simulink model "ALFlight3"  (R2019a)
settings: Solver=VariableStepAuto  StartTime=0.0  StopTime=100  RelTol=1e-3
InitFcn:
  | Ts=.05
  | load('goodMPC.mat')
  | %load('fault2mpc.mat')
  | global counts
  | counts=0
  | 
  | An=[-0.0220400000000000,0.00142200000000000,0,-32.1700000000000,0,0,0,0,0,0;-0.0575900000000000,-0.394300000000000,871,0,0,0,0,0,0,0;-9.50000000000000e-05,-0.00179300000000000,-0.546800000000000,0,0,0,0,0,0,0;0,0,1,0,0,0,0,0,0,0;0,0,0,0,-0.0639900000000000,0,-1,0.0369100000000000,0,0;0,0,0,0,-2.11100000000000,-0.504800000000000,0.193000000000000,0,0,0;0,0,0,0,0.773200000000000,0.0108700000000000,-0.179400000000000,0,0,0;0,0,0,0,0,1,0,0,0,0;0,0,0,0,0,0,1,0,0,0;0,1,0,0,0,0,0,0,0,0]
  | Bn=[0,1.91000000000000e-05,0,0;-18.5800000000000,0,0,0;-1.20000000000000,0,0,0;0,0,0,0;0,0,0,0.00839000000000000;0,0,0.184800000000000,0.105600000000000;0,0,-0.00869900000000000,-0.459100000000000;0,0,0,0;0,0,0,0;0,0,0,0]
  | 
  | load('finalWorkspace.mat')
  |  set_param('ALFlight3/ConstantA','Value','An')
  |  set_param('ALFlight3/ConstantB','Value','Bn')
model workspace (MAT data in the model file):
  MCOS : class17 (value not decoded)
values from neighbouring files (symbols this model uses):
  AfU = [-0.0194355650403 0 0.00129160400584 0 0 0 0 0 0 0 0.0910789295705 -0.529233298764 ... (100 elements, 10x10)]    [finalWorkspace.mat]
  BfU = [0 -0.0292332987635 -0.465820206007 0 0 0 0 0 0 0 4.775e-06 0 ... (40 elements, 10x4)]    [finalWorkspace.mat]
  Cn = [1 0 0 0 0 0 0 0 0 0 0 0 ... (40 elements, 4x10)]    [UpdatedWorkspace.mat]    (also in current2.mat; finalWorkspace.mat)
  Dn = [0 0 0 0 0 0 0 0 0 0 0 0 ... (16 elements, 4x4)]    [UpdatedWorkspace.mat]    (also in current2.mat; finalWorkspace.mat)
  p = 15    [calcVar.m]    (also in chanceConstraintProgramming4.m = [norminv(.505),norminv(.6),norminv(.7),norminv(.8),norminv(.; dynamicsEst.m)
undefined symbols (not defined in the file or in its folder): Earth, iA, lastPcov, lastu, lastx, MDscale, MVscale, nCC, nu, nud, nv, ny, nym, RMVscale, RYscale, ts, uoff, WGS84, xoff, Yscale
libraries: mpcsigdimcheck_private x26, simulink_extras x3, aerolibtransform2 x1, aerolibfltsims x1, commchan3 x1, aerolibanimutils x1
(part 2 of 2)

== matlab function ALFlight3/Plant/MATLAB Function ==
  data: nextState output; state input; y output; action input; Ts input; time input; currentState data_store_memory; counts data_store_memory; Damage data_store_memory
function [nextState,y] = fcn2(state, action,Ts,time)
global currentState
global Damage
coder.extrinsic('evalin')
coder.extrinsic('assignin')
Anominal=[-0.0220400000000000,0.00142200000000000,0,-32.1700000000000,0,0,0,0,0,0,0;
    -0.0575900000000000,-0.394300000000000,871,0,0,0,0,0,0,0,0;
    -9.50000000000000e-05,-0.00179300000000000,-0.546800000000000,0,0,0,0,0,0,0,0;
    0,0,1,0,0,0,0,0,0,0,0;
    0,0,0,0,-0.0639900000000000,0,-1,0.0369100000000000,0,0,0;
    0,0,0,0,-2.11100000000000,-0.504800000000000,0.193000000000000,0,0,0,0;
    0,0,0,0,0.773200000000000,0.0108700000000000,-0.179400000000000,0,0,0,0;
    0,0,0,0,0,1,0,0,0,0,0;
    0,0,0,0,0,0,1,0,0,0,0;
    1,0,0,0,0,0,0,0,0,0,0;
    0,1,0,0,0,0,0,0,0,0,0];
Bnominal=[0,1.91000000000000e-05,0,0;
    -18.5800000000000,0,0,0;
    -1.20000000000000,0,0,0;
    0,0,0,0;
    0,0,0,0.00839000000000000;
    0,0,0.184800000000000,0.105600000000000;
    0,0,-0.00869900000000000,-0.459100000000000;
    0,0,0,0;
    0,0,0,0;
    0,0,0,0;
    0,0,0,0];

Afault2=[-0.0220400000000000,0.00142200000000000,0,-32.1700000000000,0,0,0,0,0,0,0;
    -0.0575900000000000,-0.394300000000000,871,0,0,0,0,0,0,0,0;
    -9.50000000000000e-05,-0.00179300000000000,-0.546800000000000,0,0,0,0,0,0,0,0;
    0,0,1,0,0,0,0,0,0,0,0;
    0,0,0,0,0,-0.00110800000000000,-1,0.0369100000000000,0,0,0;
    0,0,0,0,-1.23500000000000,-0.481800000000000,0.0891100000000000,0,0,0,0;
    0,0,0,0,0,-0.0519300000000000,0,0,0,0,0;
    0,0,0,0,0,1,0,0,0,0,0;
    0,0,0,0,0,0,1,0,0,0,0;
    1,0,0,0,0,0,0,0,0,0,0;
    0,1,0,0,0,0,0,0,0,0,0];
Bfault2=[0,1.91000000000000e-05,0,0;
    -18.5800000000000,0,0,0;
    -1.20000000000000,0,0,0;
    0,0,0,0;
    0,0,0,0;
    0,0,0.187900000000000,0;
    0,0,0,0;
    0,0,0,0;
    0,0,0,0;
    0,0,0,0;
    0,0,0,0];

Afault1_2=[-0.0777422601610909,0.364315718281914,0,-49.5311012194985,0,0,0,0,0,0,0;
    0,-2.11693319505418,-8.082029025490,0,0,0,0,0,0,0,0;
    0.00516641602336364,-3.5543885272319,-2.926680000000,-2.37481704217243,0,0,0,0,0,0,0;
    0,0,1,0,0,0,0,0,0,0,0;
    0,0,0,0,-1.73568157299046,-0.00695689900121296,-246.715568807515,49.5311012194985,0,0,0;
    0,0,32.90144280000,31.3713331270978,-0.0210854784922154,-0.00633571574984461,0.00174212652554297,0,0,0,0;
    0,0,0,13.2100000000000,0.0233794202315124,-4.26083552968259e-05,-0.00576851579403181,0,0,0,0;
    0,0,0,0,0,1,0.0479459770467924,0,0,0,0;
    0,0,0,0,0,0,1,0,0,0,0;
    1,0,0,0,0,0,0,0,0,0,0;
    0,1,0,0,0,0,0,0,0,0,0]*.25
Bfault1_2=[0,0,0,0;
    -.11693319505418,0,0,0;
    -1.863280824027,0,0,0;
    0,0,0,0;
    0,0,0,-0.00412083182815909;
    0,0,0.00602442242634726,0.00602442242634726;
    0,0,0,-0.0221156677865658;
    0,0,0,0;0,0,0,0;0,0,0,0;0,0,0,0]*.25
 
Afault1=[-0.00470000000000000,-0.0107700000000000,0,-623300,0,0,0,0,0,0,0;
     -0.310000000000000,-0.253000000000000,16780000,-28300,0,0,0,0,0,0,0;
     0,0,-157900,264.600000000000,0,0,0,0,0,0,0;
     0,0,1,0,0,0,0,0,0,0,0;
     0,0,0,0,-0.0470000000000000,0,-16890000,620000,0,0,0;
     0,0,463000,-7797,-0.00160000000000000,-0.201300000000000,0.105500000000000,0,0,0,0;
     0,0,0,171900,0.000570000000000000,-0.00650000000000000,-157900,5833,0,0,0;
     0,0,0,0,0,1,0.0454100000000000,0,0,0,0;
     0,0,0,0,0,0,1,0,0,0,0;
     1,0,0,0,0,0,0,0,0,0,0;
     0,871,0,0,0,0,0,0,0,0,0];
 Bfault1=[0,0,0,0;
     13.3300000000000,0,0,0;
     -0.914700000000000,0,0,0;
     0,0,0,0;
     0,0,0,5.37700000000000;
     0,0,0.0670800000000000,0.0762900000000000;
     0,0,13.3200000000000,-0.289500000000000;
     0,0,0,0;
     0,0,0,0;
     0,0,0,0;
     0,0,0,0];
 
 
 Afault3=[-0.0220400000000000,0.00142200000000000,0,-32.1700000000000,0,0,0,0,0,0,0;-0.0575900000000000,-0.394300000000000,871,0,0,0,0,0,0,0,0;-9.50000000000000e-05,-0.00179300000000000,-0.546800000000000,0,0,0,0,0,0,0,0;0,0,1,0,0,0,0,0,0,0,0;0,0,0,0,-0.0639900000000000,0,-1,0.0369100000000000,0,0,0;0,0,0,0,-2.11100000000000,-0.504800000000000,0.193000000000000,0,0,0,0;0,0,0,0,0.773200000000000,0.0108700000000000,-0.179400000000000,0,0,0,0;0,0,0,0,0,1,0,0,0,0,0;0,0,0,0,0,0,1,0,0,0,0;1,0,0,0,0,0,0,0,0,0,0;0,1,0,0,0,0,0,0,0,0,0]
Bfault3=[0,1.91000000000000e-05,0,0;
    -18.5800000000000,0,0,0;
    -1.20000000000000,0,0,0;
    0,0,0,0;
    0,0,0,0.00839000000000000;
    0,0,0,0.105600000000000;
    0,0,0,-0.459100000000000;
    0,0,0,0;
    0,0,0,0;
    0,0,0,0;
    0,0,0,0]
 
 % C=[1,0,0,0,0,0,0,0,0,0,0;
%     0,0,0,1,0,0,0,0,0,0,0;
%     0,0,0,0,0,0,0,1,0,0,0;
%     0,0,0,0,0,0,0,0,1,0,0;
%     0,0,0,0,0,0,0,0,0,1,0;
%     0,0,0,0,0,0,0,0,0,0,1]
 %y=zeros(6,1);
deltaS=zeros(11,1)
if Damage==1
    ADamage=Afault1_2
    BDamage=Bfault1_2
    A=evalin('base','Af1')
    assignin('base','AfU',A)
    B=evalin('base','Bf1')
    assignin('base','BfU',B)
elseif Damage==2
    ADamage=Afault2
    BDamage=Bfault2 
    A=evalin('base','Af2')
    assignin('base','AfU',A)
    B=evalin('base','Bf2')
    assignin('base','BfU',B)
elseif Damage==3
    ADamage=Afault3
    BDamage=Bfault3
    A=evalin('base','Af3')
    assignin('base','AfU',A)
    B=evalin('base','Bf3')
    assignin('base','BfU',B)
else
    ADamage=Afault2
    BDamage=Bfault2
    A=evalin('base','Af2')
    assignin('base','AfU',A)
    B=evalin('base','Bf2')
    assignin('base','BfU',B)
end
    
 if time<10
     deltaS=Anominal*state*Ts+Bnominal*action*Ts;
     nextState=deltaS+state
    y=nextState
 else
     deltaS=ADamage*state*Ts+BDamage*action*Ts
     nextState=deltaS+state
     y=nextState
 end
 currentState=y
end

== matlab function ALFlight3/Error/MATLAB Function2 ==
  data: error input; counts data_store_memory
function fcn(error)
global counts
if error>.1
counts=counts+1
end

== matlab function ALFlight3/MATLAB Function3 ==
  data: outputs input; counts data_store_memory; savedOutputs data_store_memory
function saveDataOutputs(outputs)
global savedOutputs
global counts
if counts>0
savedOutputs(:,counts)=outputs
end
x=savedOutputs

== matlab function ALFlight3/State space model ==
  data: state input; nextState output; action input; Ts input; time input; action output; y output
function [nextState,action,y] = fcn(state, action, Ts,time)
Anominal=[-0.0220400000000000,0.00142200000000000,0,-32.1700000000000,0,0,0,0,0,0,0,0;-0.0575900000000000,-0.394300000000000,871,0,0,0,0,0,0,0,0,0;-9.50000000000000e-05,-0.00179300000000000,-0.546800000000000,0,0,0,0,0,0,0,0,0;0,0,1,0,0,0,0,0,0,0,0,0;0,0,0,0,-0.0639900000000000,0,-1,0.0369100000000000,0,0,0,0;0,0,0,0,-2.11100000000000,-0.504800000000000,0.193000000000000,0,0,0,0,0;0,0,0,0,0.773200000000000,0.0108700000000000,-0.179400000000000,0,0,0,0,0;0,0,0,0,0,1,0,0,0,0,0,0;0,0,0,0,0,0,1,0,0,0,0,0;1,0,0,0,0,0,0,0,0,0,0,0;0,1,0,0,0,0,0,0,0,0,0,0;0,0,0,0,0,0,0,0,0,0,0,0]
Bnominal=[0,1.91000000000000e-05,0,0;-18.5800000000000,0,0,0;-1.20000000000000,0,0,0;0,0,0,0;0,0,0,0.00839000000000000;0,0,0.184800000000000,0.105600000000000;0,0,-0.00869900000000000,-0.459100000000000;0,0,0,0;0,0,0,0;0,0,0,0;0,0,0,0;0,0,0,0]

Afault2=[-0.0220400000000000,0.00142200000000000,0,-32.1700000000000,0,0,0,0,0,0,0;
    -0.0575900000000000,-0.394300000000000,871,0,0,0,0,0,0,0,0;
    -9.50000000000000e-05,-0.00179300000000000,-0.546800000000000,0,0,0,0,0,0,0,0;
    0,0,1,0,0,0,0,0,0,0,0;
    0,0,0,0,0,-0.00110800000000000,-1,0.0369100000000000,0,0,0;
    0,0,0,0,-1.23500000000000,-0.481800000000000,0.0891100000000000,0,0,0,0;
    0,0,0,0,0,-0.0519300000000000,0,0,0,0,0;
    0,0,0,0,0,1,0,0,0,0,0;
    0,0,0,0,0,0,1,0,0,0,0;
    1,0,0,0,0,0,0,0,0,0,0;
    0,1,0,0,0,0,0,0,0,0,0];
Bfault2=[0,1.91000000000000e-05,0,0;
    -18.5800000000000,0,0,0;
    -1.20000000000000,0,0,0;
    0,0,0,0;
    0,0,0,0;
    0,0,0.187900000000000,0;
    0,0,0,0;
    0,0,0,0;
    0,0,0,0;
    0,0,0,0;
    0,0,0,0];
     
 Afault1=[-0.00470000000000000,-0.0107700000000000,0,-623300,0,0,0,0,0,0,0;
     -0.310000000000000,-0.253000000000000,16780000,-28300,0,0,0,0,0,0,0;
     0,0,-157900,264.600000000000,0,0,0,0,0,0,0;
     0,0,1,0,0,0,0,0,0,0,0;
     0,0,0,0,-0.0470000000000000,0,-16890000,620000,0,0,0;
     0,0,463000,-7797,-0.00160000000000000,-0.201300000000000,0.105500000000000,0,0,0,0;
     0,0,0,171900,0.000570000000000000,-0.00650000000000000,-157900,5833,0,0,0;
     0,0,0,0,0,1,0.0454100000000000,0,0,0,0;
     0,0,0,0,0,0,1,0,0,0,0;
     1,0,0,0,0,0,0,0,0,0,0;
     0,1,0,0,0,0,0,0,0,0,0];
 Bfault1=[0,0,0,0;
     13.3300000000000,0,0,0;
     -0.914700000000000,0,0,0;
     0,0,0,0;
     0,0,0,5.37700000000000;
     0,0,0.0670800000000000,0.0762900000000000;
     0,0,13.3200000000000,-0.289500000000000;
     0,0,0,0;
     0,0,0,0;
     0,0,0,0;
     0,0,0,0];
C=[1,0,0,0,0,0,0,0,0,0,0,0;0,0,0,1,0,0,0,0,0,0,0,0;0,0,0,0,0,0,0,1,0,0,0,0;0,0,0,0,0,0,0,0,1,0,0,0;0,0,0,0,0,0,0,0,0,1,0,0;0,0,0,0,0,0,0,0,0,0,1,0]
y=zeros(6,1);
deltaS=zeros(12,1)
 if time<20
     deltaS=Anominal*state*.05+Bnominal*action*.05;
    nextState=(deltaS+state);
    y=C*nextState;
 else
     nextState=zeros(12,1)
%     deltaS=Afault2*state*Ts+Bfault2*action*Ts;
%     nextState=(deltaS+state);
%     y=C*nextState;
end
end

== matlab function ALFlight3/Switch /MATLAB Function4 ==
  data: a output; actionMPC input; actionAL input; counts data_store_memory; uncertainty data_store_memory; useMPC data_store_memory; ABestGuess data_store_memory
function a = switching(actionMPC,actionAL)
coder.extrinsic('evalin')
coder.extrinsic('assignin')
coder.extrinsic('set_param')
global counts
global uncertainty
global useMPC
global ABestGuess

Anominal=[-0.0220400000000000,0.00142200000000000,0,-32.1700000000000,0,0,0,0,0,0,0;
    -0.0575900000000000,-0.394300000000000,871,0,0,0,0,0,0,0,0;
    -9.50000000000000e-05,-0.00179300000000000,-0.546800000000000,0,0,0,0,0,0,0,0;
    0,0,1,0,0,0,0,0,0,0,0;
    0,0,0,0,-0.0639900000000000,0,-1,0.0369100000000000,0,0,0;
    0,0,0,0,-2.11100000000000,-0.504800000000000,0.193000000000000,0,0,0,0;
    0,0,0,0,0.773200000000000,0.0108700000000000,-0.179400000000000,0,0,0,0;
    0,0,0,0,0,1,0,0,0,0,0;
    0,0,0,0,0,0,1,0,0,0,0;
    1,0,0,0,0,0,0,0,0,0,0;
    0,1,0,0,0,0,0,0,0,0,0];
Bnominal=[0,1.91000000000000e-05,0,0;
    -18.5800000000000,0,0,0;
    -1.20000000000000,0,0,0;
    0,0,0,0;
    0,0,0,0.00839000000000000;
    0,0,0.184800000000000,0.105600000000000;
    0,0,-0.00869900000000000,-0.459100000000000;
    0,0,0,0;
    0,0,0,0;
    0,0,0,0;
    0,0,0,0];



a=actionMPC;
if counts>3 && ~useMPC
    a=actionAL;
end
if uncertainty<.1
    useMPC=true
    
    
    Af=ABestGuess(5:15,:)*Anominal
    Af(abs(Af)<8e-5)=0
    AfU=Af([1 2 3 4 5 6 7 8 9 11],[1 2 3 4 5 6 7 8 9 11])
    Bf= ABestGuess(1:4,:)'+ABestGuess(5:15,:)'*Bnominal
    Bf(abs(Bf)<1e-5)=0
    BfU=Bf([1 2 3 4 5 6 7 8 9 11],:)

    Af2=evalin('base','Af2')
    Bf2=evalin('base','Bf2')
    
    
    set_param('ALFlight3/ConstantA','Value','AfU')
    set_param('ALFlight3/ConstantB','Value','BfU')

end
%     fault1MPC.Model.Plant.A=A
%     fault1MPC.Model.Plant.B=B
%     
%     fault2MPC.Model.Plant.A=A
%     fault2MPC.Model.Plant.B=B
%     
%     fault3MPC.Model.Plant.A=A
%     fault3MPC.Model.Plant.B=B
% set_param('testMPC/MPCController1','mpcobj','fault2MPC')

% a=actionMPC;
% if time>1000
%     a=actionAL;
% end

== matlab function ALFlight3/MATLAB Function5 ==
  data: inputs input; savedInputs data_store_memory; counts data_store_memory
function saveDataInputs(inputs)
global savedInputs
global counts
if counts>0
savedInputs(:,counts)=inputs
end
x=savedInputs

== matlab function ALFlight3/Update Plant Model ==
  data: Ac input; Bc input; Cc input; Dc input; u input; A output size=[10,10]; x input size=[11,1]; B output size=[10,4]; C output size=[4,10]; D output size=[4,4]; u output; Y output size=[4,1]; X output size=[10,1]; DX output size=[10,1]
function [A,B,C,D,u,Y,X,DX] = fcn(Ac,Bc,Cc,Dc,u,x)
% Sample time
Ts = 0.05;
x=[x(1:9);x(11)]
% Model parameters


% Continuous-time model
Ac = Ac
Bc =  Bc  
Cc = Cc
Dc = Dc

% Generate discrete-time model
nx = size(Ac,1);
nu = size(Bc,2);
M = expm([[Ac Bc]*Ts; zeros(nu,nx+nu)]);
A = M(1:nx,1:nx);
B = M(1:nx,nx+1:nx+nu);
C = Cc;
D = Dc;

% Nominal conditions for discrete-time plant
X = x;
U = u;
Y = C*x + D*u;
DX = A*x+B*u-x;

== matlab function ALFlight3/Adaptive MPC Controller/MPC/optimizer/FixedHorizonOptimizer ==
  settings: updateMethod=DISCRETE  sampleTime=ts
  data: xk1 output BlockDataType; xk input BlockDataType; old_u input BlockDataType; ym input BlockDataType; ref input BlockDataType; md input BlockDataType; umin input BlockDataType; umax input BlockDataType; ymin input BlockDataType; ymax input BlockDataType; E input BlockDataType; F input BlockDataType; G input BlockDataType; S input BlockDataType; switch_in input BlockDataType; ext_mv input BlockDataType; MVtarget input BlockDataType; isQP parameter boolean; nx parameter BlockDataType; nxp parameter BlockDataType; nup parameter BlockDataType; nu parameter BlockDataType; ny parameter BlockDataType; degrees parameter BlockDataType; Hinv parameter BlockDataType; Kx parameter BlockDataType; Ku1 parameter BlockDataType; Kut parameter BlockDataType; Kr parameter BlockDataType; Kv parameter BlockDataType; Mlim parameter BlockDataType; Mx parameter BlockDataType; Mu1 parameter BlockDataType; Mv parameter BlockDataType; z_degrees parameter BlockDataType; utarget parameter BlockDataType; p parameter BlockDataType; maxiter parameter BlockDataType; CustomSolver parameter boolean; CustomSolverCodeGen parameter boolean; UseWarmStart parameter boolean; UseSuboptimalSolution parameter boolean; nxQP parameter BlockDataType; openloopflag parameter boolean; no_umin parameter BlockDataType; no_umax parameter BlockDataType; no_ymin parameter BlockDataType; no_ymax parameter BlockDataType; switch_inport parameter BlockDataType; no_switch parameter BlockDataType; enable_value parameter BlockDataType; return_cost parameter BlockDataType; H parameter BlockDataType; return_mvseq parameter BlockDataType; return_xseq parameter BlockDataType; return_ovseq parameter BlockDataType; Linv parameter BlockDataType; Ac parameter BlockDataType; ywt input BlockDataType; uwt input BlockDataType; duwt input BlockDataType; rhoeps input BlockDataType; isLTV parameter boolean; a input BlockDataType; b input BlockDataType; c input BlockDataType; d input BlockDataType; U input BlockDataType; Y input BlockDataType; X input BlockDataType; DX input BlockDataType; Pk input BlockDataType; iA input boolean; u output BlockDataType; cost output BlockDataType; useq output BlockDataType; xseq output BlockDataType; yseq output BlockDataType; status output BlockDataType; xest output BlockDataType; Pk1 output BlockDataType; no_ywt parameter BlockDataType; no_uwt parameter BlockDataType; no_duwt parameter BlockDataType; no_rhoeps parameter BlockDataType; Wy parameter BlockDataType; Wdu parameter BlockDataType; Jm parameter BlockDataType; SuJm parameter BlockDataType; Su1 parameter BlockDataType; Sx parameter BlockDataType; Hv parameter BlockDataType; Wu parameter BlockDataType; I1 parameter BlockDataType; iAout output boolean; A parameter BlockDataType; C parameter BlockDataType; B parameter BlockDataType; D parameter BlockDataType; Cid parameter BlockDataType; Did parameter BlockDataType; Mrows parameter BlockDataType; nCC parameter BlockDataType; Ecc parameter BlockDataType; Fcc parameter BlockDataType; Scc parameter BlockDataType; Gcc parameter BlockDataType; nv parameter BlockDataType; no_md parameter BlockDataType; no_ref parameter BlockDataType; no_uref parameter BlockDataType; no_mv parameter BlockDataType; RYscale parameter BlockDataType; RMDscale parameter BlockDataType; myindex parameter BlockDataType; xoff parameter BlockDataType; CustomEstimation parameter boolean; mvindex parameter BlockDataType; mdindex parameter BlockDataType; unindex parameter BlockDataType; nxid parameter BlockDataType; Uscale parameter BlockDataType; Yscale parameter BlockDataType; uoff parameter BlockDataType; voff parameter BlockDataType; yoff parameter BlockDataType; myoff parameter BlockDataType; no_cc parameter BlockDataType
function [xk1, u, cost, useq, xseq, yseq, status, xest, Pk1, iAout] = fcn(...
            xk, old_u, ym, ref, md, umin, umax, ymin, ymax, E, F, G, S,...
            switch_in, ext_mv, MVtarget, isQP, nx, nxp, nup, ...
            nu, ny, degrees, Hinv, Kx, Ku1, Kut, Kr, Kv, Mlim, ...
            Mx, Mu1, Mv, z_degrees, utarget, p, maxiter, ...
            CustomSolver, CustomSolverCodeGen, UseWarmStart, UseSuboptimalSolution, nxQP, openloopflag, ...
            no_umin, no_umax, no_ymin, no_ymax, switch_inport, no_switch, enable_value, ...
            return_cost, H, return_mvseq, return_xseq, return_ovseq, Linv, Ac, ...
            ywt, uwt, duwt, rhoeps, isLTV, a, b, c, d, U, Y, X, DX, Pk, iA, ...
            no_ywt, no_uwt, no_duwt, no_rhoeps,...
            Wy, Wdu, Jm, SuJm, Su1, Sx, Hv, Wu, I1, ...
            A, C, B, D, Cid, Did, Mrows, nCC, Ecc, Fcc, Scc, Gcc, ...
            nv, no_md, no_ref, no_uref, no_mv, RYscale, RMDscale, myindex, ...
            xoff, CustomEstimation, mvindex, mdindex, unindex, nxid, Uscale, Yscale, uoff, voff, yoff, myoff, no_cc)
%#codegen
coder.extrinsic('mpcblock_optimizer_double_mex');
coder.extrinsic('mpcblock_optimizer_single_mex');
coder.extrinsic('mpcblock_refmd_double_mex');
coder.extrinsic('mpcblock_refmd_single_mex');

% Constants
isSimulation = coder.target('Sfun') && ~coder.target('RtwForRapid') && ~coder.target('RtwForSim');
isAdaptive = ~isLTV; % isLTV=true forces isAdaptive=false
isDouble = isa(ref,'double');
if isDouble
    DataType = 'double';
else
    DataType = 'single';
end
ZERO = zeros('like',ref);
ONE = ones('like',ref);
hasMD = nv>1;

% Pre-allocate all the MEX block outputs for the simulation mode
%#ok<*NASGU>
if isSimulation
    rseq = zeros(p*ny,1,'like',ref); %#ok<*NASGU>
    vseq = zeros((p+1)*nv,1,'like',ref);
    v = zeros(nv,1,'like',ref);
    xk1 = zeros(nx,1,'like',ref);
    u = zeros(nu,1,'like',ref);
    cost = ZERO;
    useq = zeros(p+1,nu,'like',ref); %#ok<*PREALL>
    status = ONE;
    xest = zeros(nx,1,'like',ref);
    iAout = iA;
end

% Model update
nym = length(myindex);
ai=zeros(nxp,nxp,'like',ref);
bi=zeros(nxp,nup,'like',ref);
ci=zeros(ny,nxp,'like',ref);
di=zeros(ny,nup,'like',ref);

ai(:,:)=a(:,:,1);
bi(:,:)=b(:,:,1);
ci(:,:)=c(:,:,1);
di(:,:)=d(:,:,1);

% Allocate matrices. Must allocate 3D matrix also in Adaptive case,
% otherwise EML code does not compile.
Bu=zeros(nx,nu,p+1,'like',ref);
Bv=zeros(nx,nv,p+1,'like',ref);
Dv=zeros(ny,nv,p+1,'like',ref);
Dvm=zeros(nym,nv,p+1,'like',ref);
Cm=zeros(nym,nx,p+1,'like',ref);
if ~isLTV
    % Adaptive
    [A(:,:,1),C(:,:,1),Bu(:,:,1),Bv(:,:,1),Cm(:,:,1),Dv(:,:,1),Dvm(:,:,1),Qk,Rk,Nk] = mpc_plantupdate(...
        ai,bi,ci,di,A(:,:,1),B(:,:,1),C(:,:,1),D(:,:,1),mvindex,mdindex,unindex,nxp,nup,ny,nv,nxid, ...
        myindex,Uscale,Yscale,Cid,Did);
else
    % Retrieve LTV model
    for i=1:p+1
        ai(1:nxp,1:nxp)=a(:,:,i);
        bi(1:nxp,1:nup)=b(:,:,i);
        ci(1:ny,1:nxp)=c(:,:,i);
        di(1:ny,1:nup)=d(:,:,i);
        [A(:,:,i),C(:,:,i),Bu(:,:,i),Bv(:,:,i),Cm(:,:,i),Dv(:,:,i),Dvm(:,:,i),Qk,Rk,Nk] =...
            mpc_plantupdate(ai,bi,ci,di,A(:,:,i),B(:,:,i),C(:,:,i),D(:,:,i),mvindex,mdindex,unindex,nxp,nup,ny,nv,nxid, ...
            myindex,Uscale,Yscale,Cid,Did);
    end
end

% Offset update together with Mlim, utarget, Bv and Dv values
[Mlim, utarget, uoff, voff, yoff, myoff, xoff, Bv, Dv] = ...
    mpc_updateFromNominal(isAdaptive,isQP,p,Mlim,Mrows,...
       U,Uscale,uoff,mvindex,voff,mdindex,utarget,nu,nv-1,...
       Y,Yscale,yoff,myoff,myindex,ny,...
       X,xoff,nxp,DX,A,Bu,Bv,C,Dv,nCC);

% Remove last u offset
old_u = old_u - uoff;       

% Get reference and MD signals -- accounting for previewing
if isSimulation
    if isDouble
        [rseq, vseq, v] = mpcblock_refmd_double_mex(ref,md,nv,ny,p,yoff,voff,no_md,no_ref,openloopflag, RYscale, RMDscale);
    else
        [rseq, vseq, v] = mpcblock_refmd_single_mex(ref,md,nv,ny,p,yoff,voff,no_md,no_ref,openloopflag, RYscale, RMDscale);        
    end
else
    % When doing code generation, use M code directly
    [rseq, vseq, v] = mpcblock_refmd(ref,md,nv,ny,p,yoff,voff,no_md,no_ref,openloopflag, RYscale, RMDscale);
end

% External MV override.  
% NOTE: old_u and ext_mv input signals are dimensionless and offset-free.
if no_mv==ONE
    % no external mv: old_u is the optimal u[k-1] from last_mv
    delmv = zeros(nu,1,'like',ref);
else
    % has external mv: old_u is the external u[k-1]
    ext_mv = ext_mv - uoff;     % bias correction
    delmv = ext_mv - old_u;
    old_u = ext_mv;
end

% Obtain x[k|k]
xk = xk - xoff;     % Remove offset
if CustomEstimation==ONE
    % Input is x(k|k)
    xest = xk;
else
    % Calculate gain matrices, and perform measurement update.
    Kinv = eye(nym,'like',ref)/(Cm(:,:,1)*Pk*Cm(:,:,1)' + Rk);
    L = (A(:,:,1)*Pk*Cm(:,:,1)' + Nk)*Kinv;
    M = Pk*Cm(:,:,1)'*Kinv;
    % LTVKF state estimation.
    % Scale measured output and remove offset.
    ym = ym.*RYscale(myindex) - myoff;
    % Correct x(k|k-1) for possible external mv override.
    % NOTE:  Offset was removed from x[k|k-1] at k=0.
    xk = xk + Bu(:,:,1)*delmv;
    % Measurement upate to x(k|k)
    ym_est = Cm(:,:,1)*xk + Dvm(:,:,1)*v;
    y_innov = ym - ym_est;
    xest = xk + M*y_innov;
end

% Real-time MV target override
% Note: utargetValue is a vector length p*nu.  
if no_uref==ONE
    % no external utarget
    utargetValue = utarget;
else
    % Define constant targets for the entire horizon.
    MVtarget = MVtarget - uoff;         % Bias correction
    utargetValue = reshape(MVtarget(:,ones(p,1)),nu*p,1);
end

% Real-time custom constraint override (scaled E/F/S)
if no_cc~=ONE
    Ecc = E;
    Fcc = F;
    Gcc = G;
    if nv>1
        Scc = S;
    end
end

return_sequence = (return_mvseq || return_xseq || return_ovseq)*ONE;
if isSimulation
    if isDouble
        [u, cost, useq, status, iAout] = mpcblock_optimizer_double_mex(...
            rseq, vseq, umin, umax, ymin, ymax, switch_in, xest, old_u, iA, ...
            isQP, nu, ny, degrees, Hinv, Kx, Ku1, Kut, Kr, Kv, Mlim, ...
            Mx, Mu1, Mv, z_degrees, utargetValue, p, uoff, voff, yoff, maxiter, ...
            CustomSolver, false, UseWarmStart, UseSuboptimalSolution, nxQP, openloopflag, ...
            no_umin, no_umax, no_ymin, no_ymax, no_cc, switch_inport, ...
            no_switch, enable_value, return_cost, H, return_sequence, Linv, Ac, ...
            ywt, uwt, duwt, rhoeps, no_ywt, no_uwt, no_duwt, no_rhoeps,...
            Wy, Wdu, Jm, SuJm, Su1, Sx, Hv, Wu, I1, ...
            isAdaptive, isLTV, A, Bu, Bv, C, Dv, ...
            Mrows, nCC, Ecc, Fcc, Scc, Gcc);    
    else
        [u, cost, useq, status, iAout] = mpcblock_optimizer_single_mex(...
            rseq, vseq, umin, umax, ymin, ymax, switch_in, xest, old_u, iA, ...
            isQP, nu, ny, degrees, Hinv, Kx, Ku1, Kut, Kr, Kv, Mlim, ...
            Mx, Mu1, Mv, z_degrees, utargetValue, p, uoff, voff, yoff, maxiter, ...
            CustomSolver, false, UseWarmStart, UseSuboptimalSolution, nxQP, openloopflag, ...
            no_umin, no_umax, no_ymin, no_ymax, no_cc, switch_inport, ...
            no_switch, enable_value, return_cost, H, return_sequence, Linv, Ac, ...
            ywt, uwt, duwt, rhoeps, no_ywt, no_uwt, no_duwt, no_rhoeps,...
            Wy, Wdu, Jm, SuJm, Su1, Sx, Hv, Wu, I1, ...
            isAdaptive, isLTV, A, Bu, Bv, C, Dv, ...
            Mrows, nCC, Ecc, Fcc, Scc, Gcc);    
    end
else
    % When doing code generation, use M code directly
        [u, cost, useq, status, iAout] = mpcblock_optimizer(...
            rseq, vseq, umin, umax, ymin, ymax, switch_in, xest, old_u, iA, ...
            isQP, nu, ny, degrees, Hinv, Kx, Ku1, Kut, Kr, Kv, Mlim, ...
            Mx, Mu1, Mv, z_degrees, utargetValue, p, uoff, voff, yoff, maxiter, ...
            false, CustomSolverCodeGen, UseWarmStart, UseSuboptimalSolution, nxQP, openloopflag, ...
            no_umin, no_umax, no_ymin, no_ymax, no_cc, switch_inport, ...
            no_switch, enable_value, return_cost, H, return_sequence, Linv, Ac, ...
            ywt, uwt, duwt, rhoeps, no_ywt, no_uwt, no_duwt, no_rhoeps,...
            Wy, Wdu, Jm, SuJm, Su1, Sx, Hv, Wu, I1, ...
            isAdaptive, isLTV, A, Bu, Bv, C, Dv, ...
            Mrows, nCC, Ecc, Fcc, Scc, Gcc);    
end

if return_xseq || return_ovseq
    [yseq, xseq] = mpc_computeSequence(isLTV, xest, useq, vseq, uoff, yoff, xoff, p, ny, nxQP, nv, A, Bu, Bv, C, Dv);
else
    yseq = zeros(p+1,ny,'like',rseq);
    xseq = zeros(p+1,nxQP,'like',rseq);
end

if CustomEstimation==ONE
    xk1 = zeros(nx,1,'like',ref);
    Pk1 = Pk;
else
    % LTVKF state and covariance update
    xk1 = A(:,:,1)*xk + Bu(:,:,1)*(u - uoff) + Bv(:,:,1)*v + L*y_innov;
    Pk1 = A(:,:,1)*Pk*A(:,:,1)' - (A(:,:,1)*Pk*Cm(:,:,1)' + Nk)*L' + Qk;
    Pk1 = 0.5*(Pk1 + Pk1'); % guarantee symmetric for numerical stability
end
xk1 = xk1 + xoff;   % Updated state must include offset

% return xest in original value
xest = xest + xoff;

== matlab function ALFlight3/Adaptive MPC Controller/MPC/optimizer/VariableHorizonOptimizer ==
  settings: updateMethod=DISCRETE  sampleTime=ts
  data: xk1 output BlockDataType; xk input BlockDataType; old_u input BlockDataType; ym input BlockDataType; ref input BlockDataType; md input BlockDataType; umin input BlockDataType; umax input BlockDataType; ymin input BlockDataType; ymax input BlockDataType; E input BlockDataType; F input BlockDataType; G input BlockDataType; S input BlockDataType; switch_in input BlockDataType; ext_mv input BlockDataType; MVtarget input BlockDataType; isQP parameter boolean; nx parameter BlockDataType; nxp parameter BlockDataType; nup parameter BlockDataType; nu parameter BlockDataType; ny parameter BlockDataType; degrees parameter BlockDataType; Mlim parameter BlockDataType; Mx parameter BlockDataType; Mu1 parameter BlockDataType; Mv parameter BlockDataType; utarget parameter BlockDataType; p parameter BlockDataType; maxiter parameter BlockDataType; CustomSolver parameter boolean; CustomSolverCodeGen parameter boolean; UseSuboptimalSolution parameter boolean; nxQP parameter BlockDataType; openloopflag parameter boolean; no_umin parameter BlockDataType; no_umax parameter BlockDataType; no_ymin parameter BlockDataType; no_ymax parameter BlockDataType; switch_inport parameter BlockDataType; no_switch parameter BlockDataType; enable_value parameter BlockDataType; return_cost parameter BlockDataType; H parameter BlockDataType; return_mvseq parameter BlockDataType; return_xseq parameter BlockDataType; return_ovseq parameter BlockDataType; Ac parameter BlockDataType; ywt input BlockDataType; uwt input BlockDataType; duwt input BlockDataType; rhoeps input BlockDataType; isLTV parameter boolean; a input BlockDataType; b input BlockDataType; c input BlockDataType; d input BlockDataType; U input BlockDataType; Y input BlockDataType; X input BlockDataType; DX input BlockDataType; Pk input BlockDataType; iA input boolean; extp input BlockDataType; extm input BlockDataType; u output BlockDataType; cost output BlockDataType; useq output BlockDataType; xseq output BlockDataType; yseq output BlockDataType; status output BlockDataType; xest output BlockDataType; Pk1 output BlockDataType; no_ywt parameter BlockDataType; no_uwt parameter BlockDataType; no_duwt parameter BlockDataType; no_rhoeps parameter BlockDataType; Wy parameter BlockDataType; Wdu parameter BlockDataType; Wu parameter BlockDataType; iAout output boolean; A parameter BlockDataType; C parameter BlockDataType; B parameter BlockDataType; D parameter BlockDataType; Cid parameter BlockDataType; Did parameter BlockDataType; Mrows parameter BlockDataType; nCC parameter BlockDataType; Ecc parameter BlockDataType; Fcc parameter BlockDataType; Scc parameter BlockDataType; Gcc parameter BlockDataType; nv parameter BlockDataType; no_md parameter BlockDataType; no_ref parameter BlockDataType; no_uref parameter BlockDataType; no_mv parameter BlockDataType; RYscale parameter BlockDataType; RMDscale parameter BlockDataType; myindex parameter BlockDataType; xoff parameter BlockDataType; CustomEstimation parameter boolean; mvindex parameter BlockDataType; mdindex parameter BlockDataType; unindex parameter BlockDataType; nxid parameter BlockDataType; Uscale parameter BlockDataType; Yscale parameter BlockDataType; uoff parameter BlockDataType; voff parameter BlockDataType; yoff parameter BlockDataType; myoff parameter BlockDataType; no_cc parameter BlockDataType; p0 parameter
function [xk1, u, cost, useq, xseq, yseq, status, xest, Pk1, iAout] = fcn(...
            xk, old_u, ym, ref, md, umin, umax, ymin, ymax, E, F, G, S,...
            switch_in, ext_mv, MVtarget, isQP, nx, nxp, nup, ...
            nu, ny, degrees, Mlim, ...
            Mx, Mu1, Mv, utarget, p, maxiter, ...
            CustomSolver, CustomSolverCodeGen, UseSuboptimalSolution, nxQP, openloopflag, ...
            no_umin, no_umax, no_ymin, no_ymax, switch_inport, no_switch, enable_value, ...
            return_cost, H, return_mvseq, return_xseq, return_ovseq, Ac, ...
            ywt, uwt, duwt, rhoeps, isLTV, a, b, c, d, U, Y, X, DX, Pk, iA, extp, extm, ...
            no_ywt, no_uwt, no_duwt, no_rhoeps,...
            Wy, Wdu, Wu, A, C, B, D, Cid, Did, Mrows, nCC, Ecc, Fcc, Scc, Gcc, ...
            nv, no_md, no_ref, no_uref, no_mv, RYscale, RMDscale, myindex, ...
            xoff, CustomEstimation, mvindex, mdindex, unindex, nxid, Uscale, Yscale, uoff, voff, yoff, myoff, no_cc, ...
            p0)
%#codegen
coder.extrinsic('mpcblock_optimizerPM_double_mex');
coder.extrinsic('mpcblock_optimizerPM_single_mex');
coder.extrinsic('mpcblock_refmd_double_mex');
coder.extrinsic('mpcblock_refmd_single_mex');

% The following is for DEBUG:
%%%%%%%%%%%%%%%
% coder.extrinsic('mpcblock_optimizerPM');
%%%%%%%%%%%%%%%

% Constants
isSimulation = coder.target('Sfun') && ~coder.target('RtwForRapid') && ~coder.target('RtwForSim');
isAdaptive = ~isLTV; % isLTV=true forces isAdaptive=false
isDouble = isa(ref,'double');
if isDouble
    DataType = 'double';
else
    DataType = 'single';
end
ZERO = zeros('like',ref);
ONE = ones('like',ref);
hasMD = nv>1;

% Keep output arguments related to prediction horizon (useq,xseq,yseq) of 
% size pmax, so that they don't change dimension in case extp varies. 
% Here pmax = input parameter 'p'.

% Pre-allocate all the MEX block outputs for the simulation mode
%#ok<*NASGU>
if isSimulation
    rseq = zeros(extp*ny,1,'like',ref); %#ok<*NASGU>
    vseq = zeros((extp+1)*nv,1,'like',ref);
    v = zeros(nv,1,'like',ref);
    xk1 = zeros(nx,1,'like',ref);
    u = zeros(nu,1,'like',ref);
    cost = ZERO;
    useq = zeros(p+1,nu,'like',ref); %#ok<*PREALL>
    status = ONE;
    xest = zeros(nx,1,'like',ref);
    iAout = iA;
end

% Model update
nym = length(myindex);
ai=zeros(nxp,nxp,'like',ref);
bi=zeros(nxp,nup,'like',ref);
ci=zeros(ny,nxp,'like',ref);
di=zeros(ny,nup,'like',ref);

ai(:,:)=a(:,:,1);
bi(:,:)=b(:,:,1);
ci(:,:)=c(:,:,1);
di(:,:)=d(:,:,1);

% Allocate matrices. Must allocate 3D matrix also in Adaptive case,
% otherwise EML code does not compile.
Bu=zeros(nx,nu,extp+1,'like',ref);
Bv=zeros(nx,nv,extp+1,'like',ref);
Dv=zeros(ny,nv,extp+1,'like',ref);
Dvm=zeros(nym,nv,extp+1,'like',ref);
Cm=zeros(nym,nx,extp+1,'like',ref);
if ~isLTV
    % Adaptive
    [A(:,:,1),C(:,:,1),Bu(:,:,1),Bv(:,:,1),Cm(:,:,1),Dv(:,:,1),Dvm(:,:,1),Qk,Rk,Nk] = mpc_plantupdate(...
        ai,bi,ci,di,A(:,:,1),B(:,:,1),C(:,:,1),D(:,:,1),mvindex,mdindex,unindex,nxp,nup,ny,nv,nxid, ...
        myindex,Uscale,Yscale,Cid,Did);
else
    % Retrieve LTV model
    for i=1:extp+1
        ai(1:nxp,1:nxp)=a(:,:,i);
        bi(1:nxp,1:nup)=b(:,:,i);
        ci(1:ny,1:nxp)=c(:,:,i);
        di(1:ny,1:nup)=d(:,:,i);
        [A(:,:,i),C(:,:,i),Bu(:,:,i),Bv(:,:,i),Cm(:,:,i),Dv(:,:,i),Dvm(:,:,i),Qk,Rk,Nk] =...
            mpc_plantupdate(ai,bi,ci,di,A(:,:,i),B(:,:,i),C(:,:,i),D(:,:,i),mvindex,mdindex,unindex,nxp,nup,ny,nv,nxid, ...
            myindex,Uscale,Yscale,Cid,Did);
    end
end

% Offset update together with Mlim, utarget, Bv and Dv values
[Mlim, utarget, uoff, voff, yoff, myoff, xoff, Bv, Dv] = ...
    mpc_updateFromNominal(isAdaptive,isQP,p0,Mlim,Mrows,...
       U,Uscale,uoff,mvindex,voff,mdindex,utarget,nu,nv-1,...
       Y,Yscale,yoff,myoff,myindex,ny,...
       X,xoff,nxp,DX,A,Bu,Bv,C,Dv,nCC);

% Remove last u offset
old_u = old_u - uoff;       

% Get reference and MD signals -- accounting for previewing
if isSimulation
    if isDouble
        %%%%%%%%%%%%%%%%%%%%%%%%%%%%%%%%%%%%%%%%%%%%%
        %%%%%% TEMPORARILY DISABLE MEX FILE %%%%%%%%%
        %%%%%%%%%%%%%%%%%%%%%%%%%%%%%%%%%%%%%%%%%%%%%
        [rseq, vseq, v] = mpcblock_refmd_double_mex(ref,md,nv,ny,extp,yoff,voff,no_md,no_ref,openloopflag, RYscale, RMDscale);
        %[rseq, vseq, v] = mpcblock_refmd(ref,md,nv,ny,extp,yoff,voff,no_md,no_ref,openloopflag, RYscale, RMDscale);
    else
        %%%%%%%%%%%%%%%%%%%%%%%%%%%%%%%%%%%%%%%%%%%%%
        %%%%%% TEMPORARILY DISABLE MEX FILE %%%%%%%%%
        %%%%%%%%%%%%%%%%%%%%%%%%%%%%%%%%%%%%%%%%%%%%%
        [rseq, vseq, v] = mpcblock_refmd_single_mex(ref,md,nv,ny,extp,yoff,voff,no_md,no_ref,openloopflag, RYscale, RMDscale);        
        %[rseq, vseq, v] = mpcblock_refmd(ref,md,nv,ny,extp,yoff,voff,no_md,no_ref,openloopflag, RYscale, RMDscale);        
    end
else
    % When doing code generation, use M code directly
    [rseq, vseq, v] = mpcblock_refmd(ref,md,nv,ny,extp,yoff,voff,no_md,no_ref,openloopflag, RYscale, RMDscale);
end

% External MV override.  
% NOTE: old_u and ext_mv input signals are dimensionless and offset-free.
if no_mv==ONE
    % no external mv: old_u is the optimal u[k-1] from last_mv
    delmv = zeros(nu,1,'like',ref);
else
    % has external mv: old_u is the external u[k-1]
    ext_mv = ext_mv - uoff;     % bias correction
    delmv = ext_mv - old_u;
    old_u = ext_mv;
end

% Obtain x[k|k]
xk = xk - xoff;     % Remove offset
if CustomEstimation==ONE
    % Input is x(k|k)
    xest = xk;
else
    % Calculate gain matrices, and perform measurement update.
    Kinv = eye(nym,'like',ref)/(Cm(:,:,1)*Pk*Cm(:,:,1)' + Rk);
    L = (A(:,:,1)*Pk*Cm(:,:,1)' + Nk)*Kinv;
    M = Pk*Cm(:,:,1)'*Kinv;
    % LTVKF state estimation.
    % Scale measured output and remove offset.
    ym = ym.*RYscale(myindex) - myoff;
    % Correct x(k|k-1) for possible external mv override.
    % NOTE:  Offset was removed from x[k|k-1] at k=0.
    xk = xk + Bu(:,:,1)*delmv;
    % Measurement upate to x(k|k)
    ym_est = Cm(:,:,1)*xk + Dvm(:,:,1)*v;
    y_innov = ym - ym_est;
    xest = xk + M*y_innov;
end

% Real-time MV target override
% Note: utargetValue is a vector length p*nu.  
if no_uref==ONE
    % no external utarget
    utargetValue = utarget;
else
    % Define constant targets for the entire horizon.
    MVtarget = MVtarget - uoff;         % Bias correction
    utargetValue = reshape(MVtarget(:,ones(p,1)),nu*p,1);
end

% Real-time custom constraint override (scaled E/F/S)
if no_cc~=ONE
    Ecc = E;
    Fcc = F;
    Gcc = G;
    if nv>1
        Scc = S;
    end
end

return_sequence = (return_mvseq || return_xseq || return_ovseq)*ONE;

if numel(extm) > 1
    nMoves = numel(extm)*nu;
    %extm(end) = extp - sum(extm(1:end-1));
else
    nMoves = extm*nu;
    %extm = [ones(1,extm-1), extp-extm+1];
end
extdegrees=nMoves+isQP;
extz_degrees = zeros(extdegrees,1,'like',ref);

% The following is for DEBUG:
%%%%%%%%%%%%%%%
% u=zeros(nu,1,'like',ref);
% cost=ZERO;
% useq1=zeros(p+1,nu,'like',ref);
% status=ZERO;
% iAout=false(size(iA));
%%%%%%%%%%%%%%%

if isSimulation
    if isDouble
        %%%%%%%%%%%%%%%%%%%%%%%%%%%%%%%%%%%%%%%%%%%%%
        %%%%%% TEMPORARILY DISABLE MEX FILE %%%%%%%%%
        %%%%%%%%%%%%%%%%%%%%%%%%%%%%%%%%%%%%%%%%%%%%%
        %[u, cost, useq1, status, iAout] = mpcblock_optimizerPM(...
        [u, cost, useq1, status, iAout] = mpcblock_optimizerPM_double_mex(...
            rseq, vseq, umin, umax, ymin, ymax, switch_in, xest, old_u, iA, isQP, nu, ny, ...
            Mlim, Mx, Mu1, Mv, extz_degrees, ...
            utargetValue, extp, extm, uoff, voff, yoff, maxiter,...
            CustomSolver, false, UseSuboptimalSolution, nxQP, openloopflag,...
            no_umin, no_umax, no_ymin, no_ymax, switch_inport,...
            no_switch, enable_value, return_cost, H, return_sequence, Ac,...
            ywt, uwt, duwt, rhoeps, no_ywt, no_uwt, no_duwt, no_rhoeps,...
            Wy, Wdu, Wu, isLTV, A, Bu, Bv, C, Dv,...
            Mrows, nCC, Ecc, Fcc, Scc, Gcc,...
            p0,degrees,p);    
    else
        %%%%%%%%%%%%%%%%%%%%%%%%%%%%%%%%%%%%%%%%%%%%%
        %%%%%% TEMPORARILY DISABLE MEX FILE %%%%%%%%%
        %%%%%%%%%%%%%%%%%%%%%%%%%%%%%%%%%%%%%%%%%%%%%
        %[u, cost, useq1, status, iAout] = mpcblock_optimizerPM(...
        [u, cost, useq1, status, iAout] = mpcblock_optimizerPM_single_mex(...
            rseq, vseq, umin, umax, ymin, ymax, switch_in, xest, old_u, iA, ...
            isQP, nu, ny, Mlim, ...
            Mx, Mu1, Mv, extz_degrees, utargetValue, extp, extm, uoff, voff, yoff, maxiter, ...
            CustomSolver, false, UseSuboptimalSolution, nxQP, openloopflag, ...
            no_umin, no_umax, no_ymin, no_ymax, switch_inport, ...
            no_switch, enable_value, return_cost, H, return_sequence, Ac, ...
            ywt, uwt, duwt, rhoeps, no_ywt, no_uwt, no_duwt, no_rhoeps,...
            Wy, Wdu, Wu, isLTV, A, Bu, Bv, C, Dv, ...
            Mrows, nCC, Ecc, Fcc, Scc, Gcc, ...
            p0,degrees,p);    
    end
else
    % When doing code generation, use M code directly
        [u, cost, useq1, status, iAout] = mpcblock_optimizerPM(...
            rseq, vseq, umin, umax, ymin, ymax, switch_in, xest, old_u, iA, ...
            isQP, nu, ny, Mlim, ...
            Mx, Mu1, Mv, extz_degrees, utargetValue, extp, extm, uoff, voff, yoff, maxiter, ...
            false, CustomSolverCodeGen, UseSuboptimalSolution, nxQP, openloopflag, ...
            no_umin, no_umax, no_ymin, no_ymax, switch_inport, ...
            no_switch, enable_value, return_cost, H, return_sequence, Ac, ...
            ywt, uwt, duwt, rhoeps, no_ywt, no_uwt, no_duwt, no_rhoeps,...
            Wy, Wdu, Wu, isLTV, A, Bu, Bv, C, Dv, ...
            Mrows, nCC, Ecc, Fcc, Scc, Gcc, ...
            p0,degrees,p);
end

% Add missing zeros in useq
useq = zeros(p+1,nu,'like',rseq);
for k=1:p+1
    if k<=extp+1
        for i=1:nu
            useq(k,i)=useq1(k,i);
        end
    end
end

if return_xseq || return_ovseq
    [yseq, xseq] = mpc_computeSequence(isLTV, xest, useq, vseq, uoff, yoff, xoff, extp, ny, nxQP, nv, A, Bu, Bv, C, Dv);
else
    yseq = zeros(p+1,ny,'like',rseq);
    xseq = zeros(p+1,nxQP,'like',rseq);
end

if CustomEstimation==ONE
    xk1 = zeros(nx,1,'like',ref);
    Pk1 = Pk;
else
    % LTVKF state and covariance update
    xk1 = A(:,:,1)*xk + Bu(:,:,1)*(u - uoff) + Bv(:,:,1)*v + L*y_innov;
    Pk1 = A(:,:,1)*Pk*A(:,:,1)' - (A(:,:,1)*Pk*Cm(:,:,1)' + Nk)*L' + Qk;
    Pk1 = 0.5*(Pk1 + Pk1'); % guarantee symmetric for numerical stability
end
xk1 = xk1 + xoff;   % Updated state must include offset

% return xest in original value
xest = xest + xoff;
